simulink library "RP_Simulator_Components"  (R2018a)
settings: Solver=VariableStepAuto  StartTime=0.0  StopTime=10.0  RelTol=1e-3
undefined symbols (not defined in the file): arenaLength, arenaWidth, chassisThickness, color1, objRadius, robotColor, robotId, startPose, wheelBase, wheelRadius, width, X, Y, Z
libraries: sm_lib x131, nesl_utility x37, Contact_Forces_Lib x18, $bdroot x8, simulink x1
(part 5 of 5)

== system RP_Simulator_Components/Obstacle Arena/Floor/Grid ==
  Mesh XY-Y : sm_lib/Body Elements/Solid  InertiaType=CalculateFromGeometry  Mass=1  MassUnits=kg  CenterOfMass=[0 0 0]  CenterOfMassUnits=m  MomentsOfInertia=[1 1 1]  MomentsOfInertiaUnits=kg*m^2  ProductsOfInertia=[0 0 0]  ProductsOfInertiaUnits=kg*m^2  BasedOnType=Density  Density=1000  DensityUnits=kg/(m^3)  DoExposeReferenceFrame=on  SerializedFrames=<Frames/>  GraphicType=FromGeometry  MarkerShape=Sphere  MarkerSize=10  MarkerSizeUnits=m  GraphicVisPropType=SimpleVisualProperties  GraphicDiffuseColor=[0.5 0.5 0.5]  GraphicSpecularColor=[0.5 0.5 0.5 1.0]  GraphicAmbientColor=[0.15 0.15 0.15 1.0]  GraphicEmissiveColor=[0.0 0.0 0.0 1.0]  GraphicShininess=75  GraphicOpacity=1.0  GeometryShape=GeneralExtrusion  RectangleSize=[1 1]  RectangleSizeUnits=m  BrickDimensions=[1 1 1]  BrickDimensionUnits=m  CylinderRadius=1  CylinderRadiusUnits=m  CylinderLength=1  CylinderLengthUnits=m  SphereRadius=1  SphereRadiusUnits=m  EllipsoidRadii=[1 1 1]  EllipsoidRadiiUnits=m  ExtrusionCrossSection=mesh_xsec  ExtrusionCrossSectionUnits=m  ExtrusionLength=grid_linewidth  ExtrusionLengthUnits=m  PolygonNumSides=3  PolygonOuterRadius=1  PolygonOuterRadiusUnits=m  ExtGeomFileType=STL  ExtGeomFileUnits=m  RevolutionCrossSection=[1 1; 1 -1; 2 -1; 2 1]  RevolutionCrossSectionUnits=m  RevolutionExtent=Full  RevolutionAngle=180  RevolutionAngleUnits=deg
  R : PMIOPort  Side=Left
  connections:
  R/RConn1 -- Mesh XY-Y/RConn1

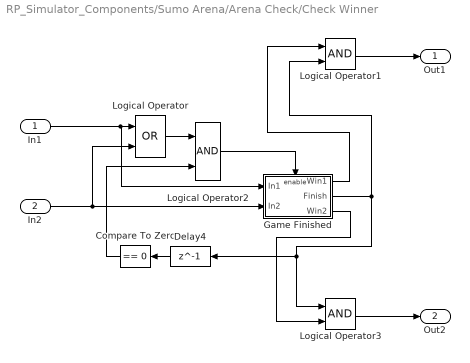
== system RP_Simulator_Components/Sumo Arena/Arena Check/Check Winner ==
  In1 : Inport
  In2 : Inport  Port=2
  Compare To Zero : simulink/Logic and Bit Operations/Compare To Zero  relop===  OutDataTypeStr=boolean
  Delay4 : Delay  DelayLength=1
  Game Finished : Subsystem  TreatAsAtomicUnit=on
  Logical Operator : Logic  Operator=OR  AllPortsSameDT=off  OutDataTypeStr=boolean
  Logical Operator1 : Logic  AllPortsSameDT=off  OutDataTypeStr=boolean
  Logical Operator2 : Logic  AllPortsSameDT=off  OutDataTypeStr=boolean
  Logical Operator3 : Logic  AllPortsSameDT=off  OutDataTypeStr=boolean
  Out1 : Outport
  Out2 : Outport  Port=2
  wires:
  Logical Operator3/1 -> Out2/1
  Game Finished/2(Finish) -> Logical Operator1/2, Delay4/1, Logical Operator3/1
  Logical Operator1/1 -> Out1/1
  In2/1 -> Game Finished/2(In2), Logical Operator/2
  Game Finished/1(Win1) -> Logical Operator1/1
  Game Finished/3(Win2) -> Logical Operator3/2
  In1/1 -> Game Finished/1(In1), Logical Operator/1
  Logical Operator/1 -> Logical Operator2/1
  Logical Operator2/1 -> Game Finished/Enable
  Compare To Zero/1 -> Logical Operator2/2
  Delay4/1 -> Compare To Zero/1

== system RP_Simulator_Components/Sumo Arena/Arena Check/Check Winner/Game Finished ==
  In1 : Inport
  In2 : Inport  Port=2
  Enable : EnablePort
  Constant : Constant
  Win1 : Outport  InitialOutput=0
  Finish : Outport  Port=2  InitialOutput=0
  Win2 : Outport  Port=3  InitialOutput=0
  wires:
  In1/1 -> Win2/1
  In2/1 -> Win1/1
  Constant/1 -> Finish/1
